simulink model "SimulacionPenduloSimpleFCN"  (R2024b)
settings: Solver=ode45  StartTime=0.0  StopTime=10  RelTol=1e-3
settings Model: Creator=Lenovo  LastModifiedBy=Lenovo

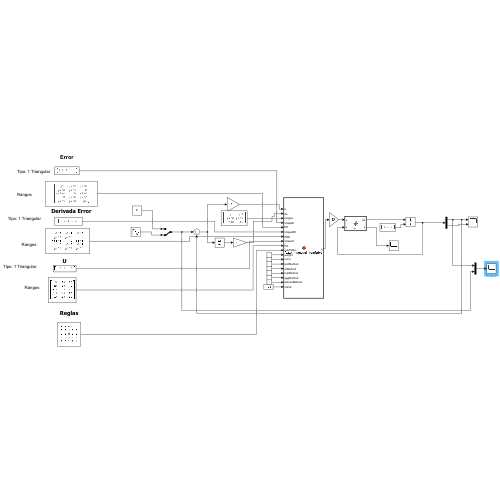
[thumbnail: Simulink's stored preview of the top-level diagram]
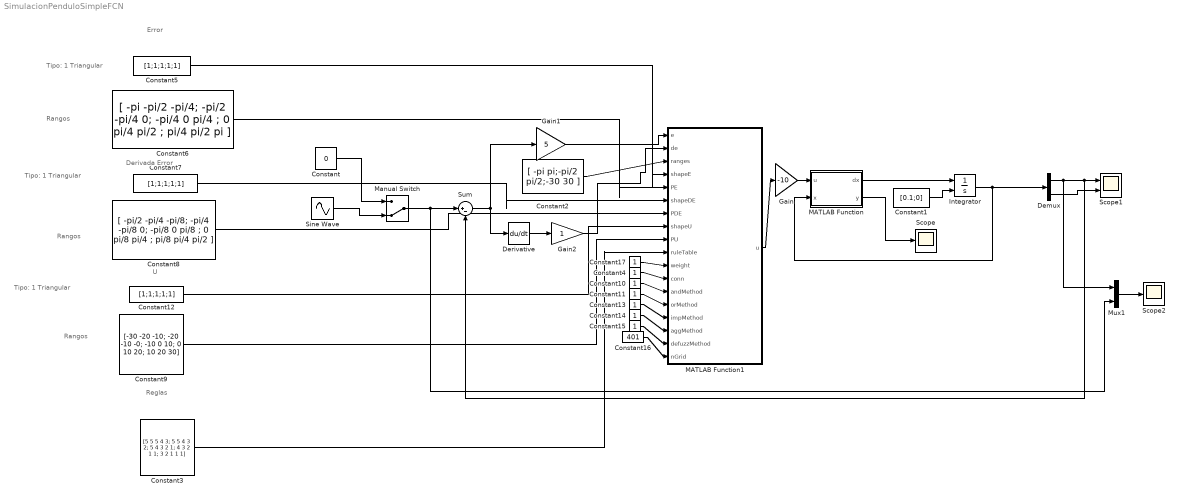
== system SimulacionPenduloSimpleFCN ==
  note: Reglas
  note: Rangos
  note: Tipo: 1 Triangular
  note: U
  note: Derivada Error
  note: Error
  note: Tipo: 1 Triangular
  note: Rangos
  note: Rangos
  note: Tipo: 1 Triangular
  Constant : Constant  Value=0
  Constant1 : Constant  Value=[0.1;0]
  Constant{4,10..11,13..15,17} (7 alike) : Constant
  Constant12 : Constant  Value=[1;1;1;1;1]
  Constant16 : Constant  Value=401
  Constant2 : Constant  Value="[ -pi   pi;-pi/2 pi/2;-30   30 ]"
  Constant3 : Constant  Value=|
      | [5 5 5 4 3;
      | 5 5 4 3 2;
      |              5 4 3 2 1;
      |              4 3 2 1 1;
      |              3 2 1 1 1]
  Constant5 : Constant  Value=[1;1;1;1;1]
  Constant6 : Constant  Value=|
      | [ -pi   -pi/2   -pi/4;
      |   -pi/2   -pi/4   0;
      |   -pi/4   0     pi/4 ;
      |    0     pi/4   pi/2 ;
      |    pi/4   pi/2    pi ]
  Constant7 : Constant  Value=[1;1;1;1;1]
  Constant8 : Constant  Value=|
      | [ -pi/2   -pi/4   -pi/8;
      |   -pi/4   -pi/8   0;
      |   -pi/8   0     pi/8 ;
      |    0     pi/8   pi/4 ;
      |    pi/8   pi/4    pi/2 ]
  Constant9 : Constant  Value=[-30 -20 -10; -20 -10 -0; -10 0 10; 0 10 20; 10 20 30]
  Demux : Demux  Outputs=2
  Derivative : Derivative
  Gain : Gain  Gain=-10
  Gain1 : Gain  Gain=5
  Gain2 : Gain
  Integrator : Integrator  InitialConditionSource=external
  MATLAB Function : MATLAB Function  TreatAsAtomicUnit=on
  MATLAB Function1 : MATLAB Function  TreatAsAtomicUnit=on
  Manual Switch : ManualSwitch  CurrentSetting=0
  Mux1 : Mux  Inputs=2
  Scope : Scope
  Scope1 : Scope  NumInputPorts=2
  Scope2 : Scope
  Sine Wave : Sin  Amplitude=.25  Frequency=4  SampleTime=0
  Sum : Sum  Inputs=|+-
  wires:
  Integrator/1 -> Demux/1, MATLAB Function/2(x)
  MATLAB Function/1(dx) -> Integrator/1
  Constant1/1 -> Integrator/2
  Demux/1 -> Mux1/1, Sum/2, Scope1/1
  Demux/2 -> Scope1/2
  MATLAB Function/2(y) -> Scope/1
  Gain/1 -> MATLAB Function/1(u)
  MATLAB Function1/1(u) -> Gain/1
  Gain1/1 -> MATLAB Function1/1(e)
  Derivative/1 -> Gain2/1
  Sum/1 -> Derivative/1, Gain1/1
  Manual Switch/1 -> Mux1/2, Sum/1
  Constant/1 -> Manual Switch/1
  Sine Wave/1 -> Manual Switch/2
  Mux1/1 -> Scope2/1
  Constant12/1 -> MATLAB Function1/8(shapeU)
  Constant7/1 -> MATLAB Function1/6(shapeDE)
  Gain2/1 -> MATLAB Function1/2(de)
  Constant2/1 -> MATLAB Function1/3(ranges)
  Constant6/1 -> MATLAB Function1/5(PE)
  Constant8/1 -> MATLAB Function1/7(PDE)
  Constant9/1 -> MATLAB Function1/9(PU)
  Constant10/1 -> MATLAB Function1/13(andMethod)
  Constant11/1 -> MATLAB Function1/14(orMethod)
  Constant13/1 -> MATLAB Function1/15(impMethod)
  Constant14/1 -> MATLAB Function1/16(aggMethod)
  Constant15/1 -> MATLAB Function1/17(defuzzMethod)
  Constant16/1 -> MATLAB Function1/18(nGrid)
  Constant4/1 -> MATLAB Function1/12(conn)
  Constant17/1 -> MATLAB Function1/11(weight)
  Constant3/1 -> MATLAB Function1/10(ruleTable)
  Constant5/1 -> MATLAB Function1/4(shapeE)

== matlab function SimulacionPenduloSimpleFCN/MATLAB Function1 ==
  data: e input; u output; de input; ranges input; shapeE input; PE input; shapeDE input; PDE input; shapeU input; PU input; ruleTable input; weight input; conn input; andMethod input; orMethod input; impMethod input; aggMethod input; defuzzMethod input; nGrid input
function u = fuzzy_mamdani_fromTable( ...
    e, de, ...
    ranges, ...
    shapeE, PE, ...
    shapeDE, PDE, ...
    shapeU, PU, ...
    ruleTable, ...
    weight, conn, ...
    andMethod, orMethod, impMethod, aggMethod, ...
    defuzzMethod, nGrid)
%#codegen
% Entradas:
%  e, de            : escalares
%  ranges           : 3x2  [emin emax; dmin dmax; umin umax]
%  shapeE/DE        : nE x 1 / nDE x 1 (1=tri,2=trap,3=gauss,4=gbell)
%  PE/PDE           : nE x 4 / nDE x 4  (rellenar con 0 si sobran)
%  shapeU           : nU x 1 (en tu caso nU=3: N,Z,P)
%  PU               : nU x 4
%  ruleTable        : nE x nDE (valores 1..nU ó -1/0/1 ó 'N/Z/P')
%  weight, conn     : escalar (peso [0,1], conn=1 AND, 2 OR)
%  andMethod        : 1=min, 2=prod
%  orMethod         : 1=max, 2=probor
%  impMethod        : 1=min, 2=prod
%  aggMethod        : 1=max, 2=probor, 3=sum (clamp a 1)
%  defuzzMethod     : 1=centroid, 2=bisector, 3=MOM, 4=SOM, 5=LOM
%  nGrid            : puntos de malla de salida

    % --- salida escalar asegurada ---
    u = 0.0;

    % --- por si llegan vectores por error ---
    if ~isscalar(e),  e  = e(1);  end
    if ~isscalar(de), de = de(1); end

    % ======== buffers fijos para no usar tamaños variables ========
    MAX_GRID = 1001;                  % sube si quieres más resolución
    yg  = zeros(1, MAX_GRID);
    agg = zeros(1, MAX_GRID);
    % ===================================================================

    % ---- universos y malla de salida (se usan los primeros N puntos) ----
    umin = ranges(3,1); umax = ranges(3,2);
    N = int32(min(max(3, round(nGrid)), MAX_GRID));
    step = (umax - umin) / double(N-1);
    for k = 1:double(N)
        yg(k) = umin + step * double(k-1);
    end

    % ---- tamaños de MFs ----
    nE  = size(PE,1);
    nDE = size(PDE,1);
    nU  = size(PU,1);     % en tu caso 3 (N,Z,P)

    % ---- fuzzificación entradas ----
    muE  = zeros(1,nE);
    muDE = zeros(1,nDE);
    for i=1:nE,   muE(i)  = evalMF(e,  shapeE(i),  PE(i,:));  end
    for i=1:nDE,  muDE(i) = evalMF(de, shapeDE(i), PDE(i,:)); end

    % ---- convertir tabla nE×nDE a reglas (iE,iDE,iU,w,conn) ----
    rules = tableToRules(ruleTable, weight, conn, nU);  % *** GENERALIZADO ***

    % ---- precalcular MFs de salida (tam fijo MAX_GRID) ----
    MUout = zeros(nU, MAX_GRID);
    for iu = 1:nU
        for k = 1:double(N)
            MUout(iu,k) = evalMF(yg(k), shapeU(iu), PU(iu,:));
        end
    end

    % ---- inferencia (implicación + agregación) ----
    R = size(rules,1);
    for r = 1:R
        iE  = rules(r,1);   iDE = rules(r,2);   iU = rules(r,3);
        w   = rules(r,4);   cn  = rules(r,5);

        a1 = muE(iE); a2 = muDE(iDE);

        % conexión
        if cn==2
            if orMethod==2
                fire = a1 + a2 - a1*a2;    % probOR
            else
                fire = max(a1,a2);         % max
            end
        else
            if andMethod==2
                fire = a1*a2;              % product
            else
                fire = min(a1,a2);         % min
            end
        end
        if fire < 0, fire = 0; elseif fire > 1, fire = 1; end
        fire = fire * max(0,min(1,w));

        % implicación y agregación
        for k = 1:double(N)
            muo = MUout(iU,k);
            if impMethod==2
                fired = muo * fire;        % product
            else
                % min
                if muo < fire, fired = muo; else, fired = fire; end
            end

            if aggMethod==3
                aggk = agg(k) + fired; if aggk > 1, aggk = 1; end
                agg(k) = aggk;
            elseif aggMethod==2
                agg(k) = agg(k) + fired - agg(k)*fired;  % probOR
            else
                if fired > agg(k), agg(k) = fired; end   % max
            end
        end
    end

    % ---- defuzzificación (siempre escalar) ----
    switch defuzzMethod
        case 2   % bisector
            Atot = 0.0;
            for k = 1:double(N-1)
                Atot = Atot + 0.5*(agg(k)+agg(k+1))*step;
            end
            if Atot <= 1e-12
                u = (umin+umax)/2;
            else
                halfA = 0.5*Atot; A = 0.0; idx = 1;
                for k = 1:double(N-1)
                    A = A + 0.5*(agg(k)+agg(k+1))*step;
                    if A >= halfA, idx = k+1; break; end
                end
                u = yg(idx);
            end

        case 3   % MOM
            m = 0.0;
            for k = 1:double(N)
                if agg(k) > m, m = agg(k); end
            end
            if m <= 1e-12
                u = (umin+umax)/2;
            else
                tol = 1e-12;
                i1 = 0; i2 = 0;
                for k = 1:double(N)
                    if (agg(k) >= m - tol), i1 = k; break; end
                end
                for k = double(N):-1:1
                    if (agg(k) >= m - tol), i2 = k; break; end
                end
                if i1==0 || i2==0, u = (umin+umax)/2;
                else, u = 0.5*(yg(i1)+yg(i2));
                end
            end

        case 4   % SOM
            m = 0.0; for k=1:double(N), if agg(k)>m, m=agg(k); end, end
            if m <= 1e-12
                u = (umin+umax)/2;
            else
                idx = 1;
                for k = 1:double(N)
                    if agg(k) >= m - 1e-12, idx = k; break; end
                end
                u = yg(idx);
            end

        case 5   % LOM
            m = 0.0; for k=1:double(N), if agg(k)>m, m=agg(k); end, end
            if m <= 1e-12
                u = (umin+umax)/2;
            else
                idx = double(N);
                for k = double(N):-1:1
                    if agg(k) >= m - 1e-12, idx = k; break; end
                end
                u = yg(idx);
            end

        otherwise  % 1: centroid
            den = 0.0; num = 0.0;
            for k = 1:double(N-1)
                den = den + 0.5*(agg(k)+agg(k+1))*step;
                num = num + 0.5*(agg(k)*yg(k) + agg(k+1)*yg(k+1))*step;
            end
            if den <= 1e-12, u = (umin+umax)/2; else, u = num/den; end
    end
end

% =================== HELPERS ===================

function rules = tableToRules(T, w, conn, nU)
    % Convierte tabla nE×nDE en matriz de reglas:
    %   [iE, iDE, iU_clamped, weight, conn]
    % Acepta T como números 1..nU, -1/0/1 ó 'N'/'Z'/'P' (se mapea a 1/2/3).
    if isstring(T) || ischar(T) || iscellstr(T)
        S = string(T); U = zeros(size(S));
        for i=1:numel(S)
            si = upper(strtrim(S(i)));
            if     si=="N", U(i)=1;
            elseif si=="Z", U(i)=2;
            elseif si=="P", U(i)=3;
            else,  U(i)=2;
            end
        end
    else
        U = double(T);
        % Soporta -1/0/1 -> 1/2/3
        if any(ismember(U,[-1 0 1])), U = (U+1) + 1; end
    end

    nE  = size(U,1);
    nDE = size(U,2);
    R   = nE*nDE;
    rules = zeros(R,5);
    k = 1;
    for iE = 1:nE
        for iDE = 1:nDE
            iU = U(iE,iDE);
            % Limita a 1..nU (en tu caso 1..3 -> N,Z,P)
            if iU < 1, iU = 1; elseif iU > nU, iU = nU; end
            rules(k,:) = [iE, iDE, iU, max(0,min(1,w)), conn];
            k = k + 1;
        end
    end
end

function mu = evalMF(x, shape, p)
    % x escalar. Formas:
    % 1=tri [a b c], 2=trap [a b c d], 3=gauss [sigma c], 4=gbell [a b c]
    if ~isscalar(x), x = x(1); end

    % Mantener 'shape' como double (no int32) para evitar conflictos de tipo
    sh = round(shape);

    % Copia de p a buffers de tamaño fijo (NO modificar 'p')
    pp4 = zeros(1,4);                    % para trap
    L   = min(numel(p),4);
    if L > 0
        pp4(1:L) = p(1:L);               % copia segura
    end

    % Para tri/gbell/gauss usamos sub-vectores de pp4
    pp3 = pp4(1:3);                      % [a b c] por defecto
    if L >= 2
        pg2 = pp4(1:2);                  % [sigma c] para gauss
    else
        pg2 = [max(pp4(1),1e-12) 0];
    end

    switch sh
        case 2  % trapezoidal [a b c d] (si faltan, d=c)
            a = pp4(1); b = pp4(2); c = pp4(3); d = pp4(4);
            if L < 4, d = c; end
            if x<=a || x>=d
                mu = 0.0;
            elseif x<b
                mu = (x-a)/(b-a+eps);
            elseif x<=c
                mu = 1.0;
            else
                mu = (d-x)/(d-c+eps);
            end

        case 3  % gauss [sigma c]
            s = max(pg2(1),1e-12); m = pg2(2);
            mu = exp(-0.5*((x-m)/s).^2);

        case 4  % gbell [a b c]
            a = max(pp3(1),1e-12); b = pp3(2); c = pp3(3);
            mu = 1.0/(1.0 + abs((x-c)/a).^(2*b));

        otherwise % 1 = triangular [a b c]
            a = pp3(1); b = pp3(2); c = pp3(3);
            if x<=a || x>=c
                mu = 0.0;
            elseif x<b
                mu = (x-a)/(b-a+eps);
            elseif x>b
                mu = (c-x)/(c-b+eps);
            else
                mu = 1.0;
            end
    end
end

== matlab function SimulacionPenduloSimpleFCN/MATLAB Function ==
  data: dx output; u input; y output; x input
function [dx, y] = fcn(u,x)

l=1; m=1; g=9.81; b=0.5; I=m*l^2;
x1=x(1);
x2=x(2);
dx1=x2;
dx2=-g/l*sin(x1)-(b*l/I)*x2+u/I;
dx = [dx1;dx2];

y = x1;
